simulink model "Ex19"  (R2019b)
settings: Solver=VariableStepAuto  StartTime=0.0  StopTime=3000  RelTol=1e-3
values from neighbouring files (symbols this model uses):
  A1 = 3.14    [Ex_19.m]
  A2 = 0.79    [Ex_19.m]
  g = 9.8    [Ex_19.m]    (also in Ex_22.m)
  Q = 0.01    [Ex_19.m]
  R1 = 10^6    (= 1000000)    [Ex_19.m]    (also in Ex_27.m = 2*qsi * sqrt(L/C); Ex_29.m = 1000)
  R2 = 2*R1    (= 2000000)    [Ex_19.m]    (also in Ex_27.m = 2 * R1; Ex_29.m = 1000000)
  rho = 1000    [Ex_19.m]
libraries: simulink_extras x2
settings Model: Creator=andre  LastModifiedBy=andre

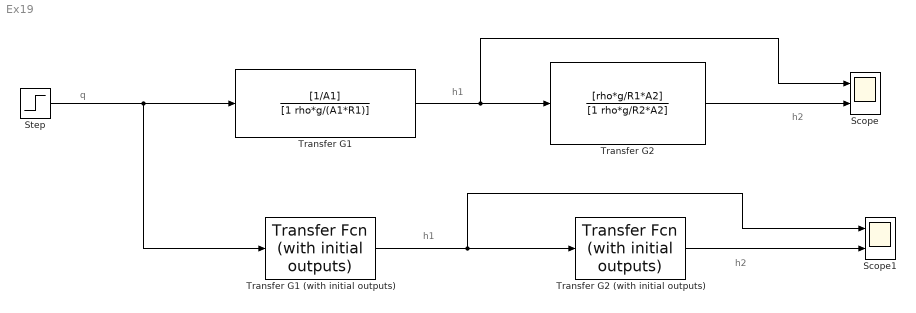
== system Ex19 ==
  note: h2
  note: h1
  note: q
  note: h2
  note: h1
  Scope : Scope  NumInputPorts=2
  Scope1 : Scope  NumInputPorts=2
  Step : Step  Time=0  After=Q  SampleTime=0
  Transfer G1 : TransferFcn  Numerator=[1/A1]  Denominator=[1 rho*g/(A1*R1)]
  Transfer G1 (with initial outputs) : simulink_extras/Additional Linear/Transfer Fcn (with initial outputs)  N=[1/A1]  D=[1 rho*g/(A1*R1)]  Y0=0.2  U0=0
  Transfer G2 : TransferFcn  Numerator=[rho*g/R1*A2]  Denominator=[1 rho*g/R2*A2]
  Transfer G2 (with initial outputs) : simulink_extras/Additional Linear/Transfer Fcn (with initial outputs)  N=[rho*g/R1*A2]  D=[1 rho*g/R2*A2]  Y0=1.0  U0=0
  wires:
  Step/1 -> Transfer G1/1, Transfer G1 (with initial outputs)/1
  Transfer G1/1 -> Scope/1, Transfer G2/1
  Transfer G2/1 -> Scope/2
  Transfer G1 (with initial outputs)/1 -> Scope1/1, Transfer G2 (with initial outputs)/1
  Transfer G2 (with initial outputs)/1 -> Scope1/2
